simulink model "DCmotormodelVuoto"  (R2024b)
settings: Solver=VariableStepAuto  StartTime=0.0  StopTime=7  MaxStep=1e-4  RelTol=1e-4  AbsTol=1e-5
values from neighbouring files (symbols this model uses):
  kt = kv    (= 0.0697098650743)    [DCMOTORELAST.m]    (also in simulazione_vuota1.mat = 0.0697; simulazione_vuota2lim.mat = 0.0697)
  kv = kvC*60/(1000*2*pi)    (= 0.0697098650743)    [DCMOTORELAST.m]    (also in simulazione_vuota1.mat = 0.0697; simulazione_vuota2lim.mat = 0.0697)
  Va = Eg+Ra*Iamax    (= 23.7583502756)    [DCMOTORELAST.m]    (also in simulazione_vuota1.mat = 23.7555140698; simulazione_vuota2lim.mat = 23.7555140698)
libraries: cstblocks x2
settings Model: Creator=marco  LastModifiedBy=david

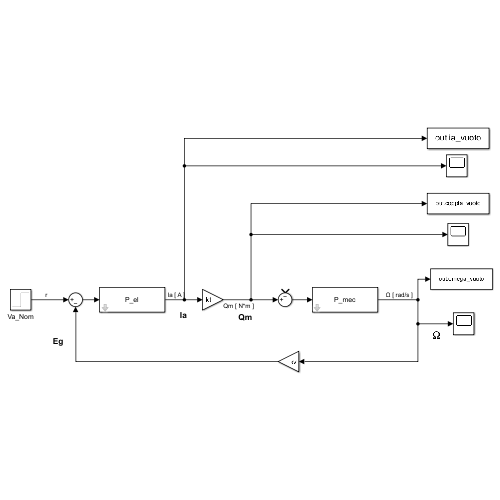
[thumbnail: Simulink's stored preview of the top-level diagram]
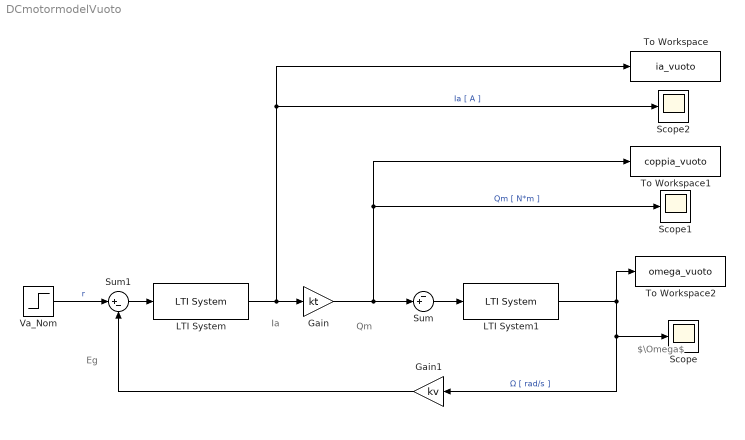
== system DCmotormodelVuoto ==
  note: $\Omega$
  note: Eg
  note: Ia
  note: Qm
  Gain : Gain  Gain=kt
  Gain1 : Gain  Gain=kv
  LTI System : cstblocks/LTI System  sys=P_el  IC=[]  PadeOrder=0
  LTI System1 : cstblocks/LTI System  sys=P_mec  IC=[]  PadeOrder=0
  Scope : Scope
  Scope1 : Scope
  Scope2 : Scope
  Sum : Sum  Inputs=-+|
  Sum1 : Sum  Inputs=|+-
  To Workspace : ToWorkspace  VariableName=ia_vuoto  SaveFormat=Timeseries  SampleTime=-1
  To Workspace1 : ToWorkspace  VariableName=coppia_vuoto  SaveFormat=Timeseries  SampleTime=-1
  To Workspace2 : ToWorkspace  VariableName=omega_vuoto  SaveFormat=Timeseries  SampleTime=-1
  Va_Nom : Step  After=Va  SampleTime=0
  wires:
  Va_Nom/1 -> Sum1/1  "r"
  LTI System/1 -> To Workspace/1, Scope2/1, Gain/1  "Ia [ A ]"
  LTI System1/1 -> Scope/1, Gain1/1, To Workspace2/1  "Ω [ rad/s ]"
  Sum1/1 -> LTI System/1
  Gain1/1 -> Sum1/2
  Sum/1 -> LTI System1/1
  Gain/1 -> To Workspace1/1, Scope1/1, Sum/2  "Qm [ N*m ]"
